simulink model "TST_ECBtn_VD"  (R2016b)
settings: Solver=FixedStepDiscrete  StartTime=0.0  StopTime=simTime  FixedStep=sampleTime  RelTol=1e-3
values from neighbouring files (symbols this model uses):
  testCase = 1    [initTST_ECBtn_VD_001.m]
libraries: simulink x4, UnitTest_Lib x2
settings Model: Creator=xinchangran  LastModifiedBy=xinchangran
settings DebuggingCC: SignalRangeChecking=error

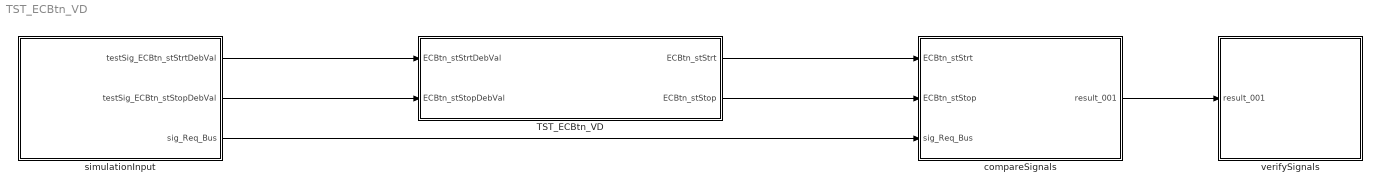
== system TST_ECBtn_VD ==
  TST_ECBtn_VD : Subsystem
  compareSignals : Subsystem
  simulationInput : Subsystem
  verifySignals : Subsystem
  wires:
  simulationInput/1(testSig_ECBtn_stStrtDebVal) -> TST_ECBtn_VD/1(ECBtn_stStrtDebVal)
  simulationInput/2(testSig_ECBtn_stStopDebVal) -> TST_ECBtn_VD/2(ECBtn_stStopDebVal)
  TST_ECBtn_VD/1(ECBtn_stStrt) -> compareSignals/1(ECBtn_stStrt)
  TST_ECBtn_VD/2(ECBtn_stStop) -> compareSignals/2(ECBtn_stStop)
  simulationInput/3(sig_Req_Bus) -> compareSignals/3(sig_Req_Bus)
  compareSignals/1(result_001) -> verifySignals/1(result_001)

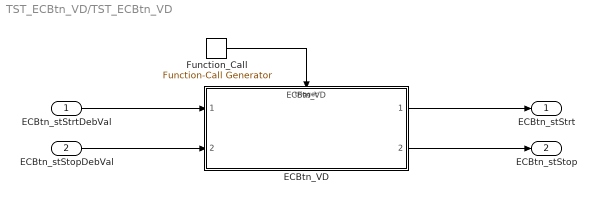
== system TST_ECBtn_VD/TST_ECBtn_VD ==
  ECBtn_stStrtDebVal : Inport
  ECBtn_stStopDebVal : Inport  Port=2
  ECBtn_VD : ModelReference  ModelNameDialog=ECBtn_VD  SimulationMode=Normal  ModelReferenceVersion=1.11  TriggerPortName=function  TriggerPortTriggerType=function-call  TriggerPortStatesWhenEnabling=held
  Function_Call : simulink/Ports & Subsystems/Function-Call Generator  sample_time=sampleTime  numberOfIterations=1
  ECBtn_stStrt : Outport
  ECBtn_stStop : Outport  Port=2
  wires:
  Function_Call/1 -> ECBtn_VD/Trigger
  ECBtn_stStrtDebVal/1 -> ECBtn_VD/1
  ECBtn_stStopDebVal/1 -> ECBtn_VD/2
  ECBtn_VD/1 -> ECBtn_stStrt/1
  ECBtn_VD/2 -> ECBtn_stStop/1

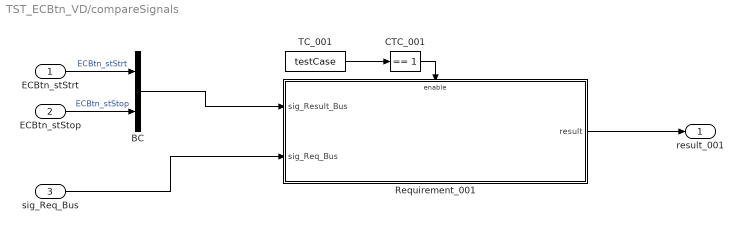
== system TST_ECBtn_VD/compareSignals ==
  ECBtn_stStrt : Inport
  ECBtn_stStop : Inport  Port=2
  sig_Req_Bus : Inport  Port=3
  BC : BusCreator  Inputs=2
  CTC_001 : simulink/Logic and Bit Operations/Compare To Constant  relop===  const=1  OutDataTypeStr=boolean
  Requirement_001 : Subsystem
  TC_001 : Constant  Value=testCase
  result_001 : Outport
  wires:
  ECBtn_stStrt/1 -> BC/1  "ECBtn_stStrt"
  ECBtn_stStop/1 -> BC/2  "ECBtn_stStop"
  TC_001/1 -> CTC_001/1
  CTC_001/1 -> Requirement_001/Enable
  sig_Req_Bus/1 -> Requirement_001/2(sig_Req_Bus)
  BC/1 -> Requirement_001/1(sig_Result_Bus)
  Requirement_001/1(result) -> result_001/1

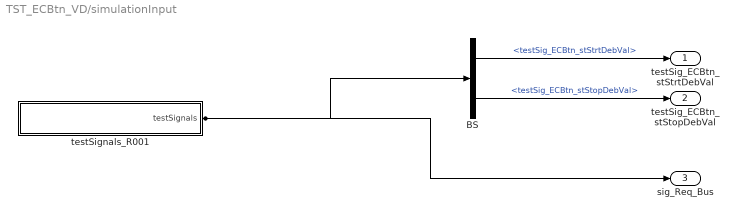
== system TST_ECBtn_VD/simulationInput ==
  BS : BusSelector  OutputSignals=testSig_ECBtn_stStrtDebVal,testSig_ECBtn_stStopDebVal
  testSignals_R001 : Subsystem
  testSig_ECBtn_stStrtDebVal : Outport
  testSig_ECBtn_stStopDebVal : Outport  Port=2
  sig_Req_Bus : Outport  Port=3
  wires:
  BS/1 -> testSig_ECBtn_stStrtDebVal/1  "<testSig_ECBtn_stStrtDebVal>"
  BS/2 -> testSig_ECBtn_stStopDebVal/1  "<testSig_ECBtn_stStopDebVal>"
  testSignals_R001/1(testSignals) -> BS/1, sig_Req_Bus/1

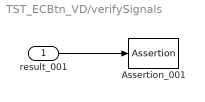
== system TST_ECBtn_VD/verifySignals ==
  result_001 : Inport
  Assertion_001 : Assertion  Enabled=off
  wires:
  result_001/1 -> Assertion_001/1

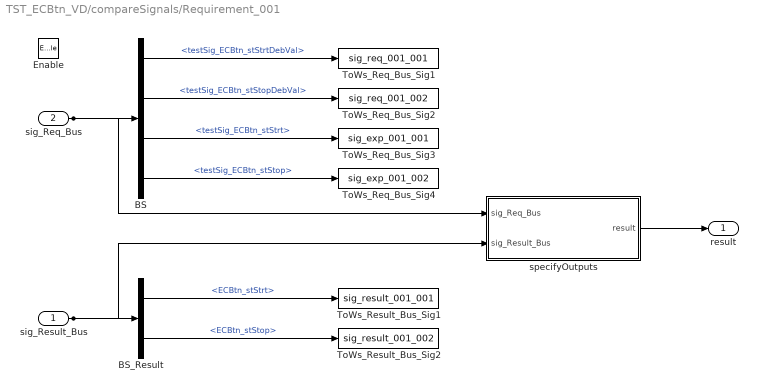
== system TST_ECBtn_VD/compareSignals/Requirement_001 ==
  sig_Result_Bus : Inport
  sig_Req_Bus : Inport  Port=2
  Enable : EnablePort
  BS : BusSelector  OutputSignals=testSig_ECBtn_stStrtDebVal,testSig_ECBtn_stStopDebVal,testSig_ECBtn_stStrt,testSig_ECBtn_stStop
  BS_Result : BusSelector  OutputSignals=ECBtn_stStrt,ECBtn_stStop
  ToWs_Req_Bus_Sig1 : ToWorkspace  VariableName=sig_req_001_001  SaveFormat=Structure With Time
  ToWs_Req_Bus_Sig2 : ToWorkspace  VariableName=sig_req_001_002  SaveFormat=Structure With Time
  ToWs_Req_Bus_Sig3 : ToWorkspace  VariableName=sig_exp_001_001  SaveFormat=Structure With Time
  ToWs_Req_Bus_Sig4 : ToWorkspace  VariableName=sig_exp_001_002  SaveFormat=Structure With Time
  ToWs_Result_Bus_Sig1 : ToWorkspace  VariableName=sig_result_001_001  SaveFormat=Structure With Time
  ToWs_Result_Bus_Sig2 : ToWorkspace  VariableName=sig_result_001_002  SaveFormat=Structure With Time
  specifyOutputs : Subsystem
  result : Outport
  wires:
  sig_Req_Bus/1 -> BS/1, specifyOutputs/1(sig_Req_Bus)
  BS/1 -> ToWs_Req_Bus_Sig1/1  "<testSig_ECBtn_stStrtDebVal>"
  BS/2 -> ToWs_Req_Bus_Sig2/1  "<testSig_ECBtn_stStopDebVal>"
  BS/3 -> ToWs_Req_Bus_Sig3/1  "<testSig_ECBtn_stStrt>"
  BS/4 -> ToWs_Req_Bus_Sig4/1  "<testSig_ECBtn_stStop>"
  sig_Result_Bus/1 -> BS_Result/1, specifyOutputs/2(sig_Result_Bus)
  BS_Result/1 -> ToWs_Result_Bus_Sig1/1  "<ECBtn_stStrt>"
  BS_Result/2 -> ToWs_Result_Bus_Sig2/1  "<ECBtn_stStop>"
  specifyOutputs/1(result) -> result/1

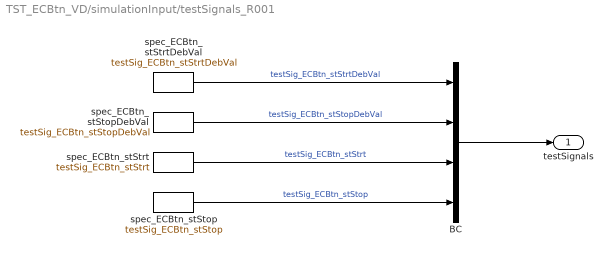
== system TST_ECBtn_VD/simulationInput/testSignals_R001 ==
  BC : BusCreator  Inputs=4
  spec_ECBtn_stStop : FromWorkspace  VariableName=testSig_ECBtn_stStop  Interpolate=off  OutputAfterFinalValue=Holding final value
  spec_ECBtn_stStopDebVal : FromWorkspace  VariableName=testSig_ECBtn_stStopDebVal  Interpolate=off  OutputAfterFinalValue=Holding final value
  spec_ECBtn_stStrt : FromWorkspace  VariableName=testSig_ECBtn_stStrt  Interpolate=off  OutputAfterFinalValue=Holding final value
  spec_ECBtn_stStrtDebVal : FromWorkspace  VariableName=testSig_ECBtn_stStrtDebVal  Interpolate=off  OutputAfterFinalValue=Holding final value
  testSignals : Outport
  wires:
  BC/1 -> testSignals/1
  spec_ECBtn_stStrtDebVal/1 -> BC/1  "testSig_ECBtn_stStrtDebVal"
  spec_ECBtn_stStopDebVal/1 -> BC/2  "testSig_ECBtn_stStopDebVal"
  spec_ECBtn_stStrt/1 -> BC/3  "testSig_ECBtn_stStrt"
  spec_ECBtn_stStop/1 -> BC/4  "testSig_ECBtn_stStop"

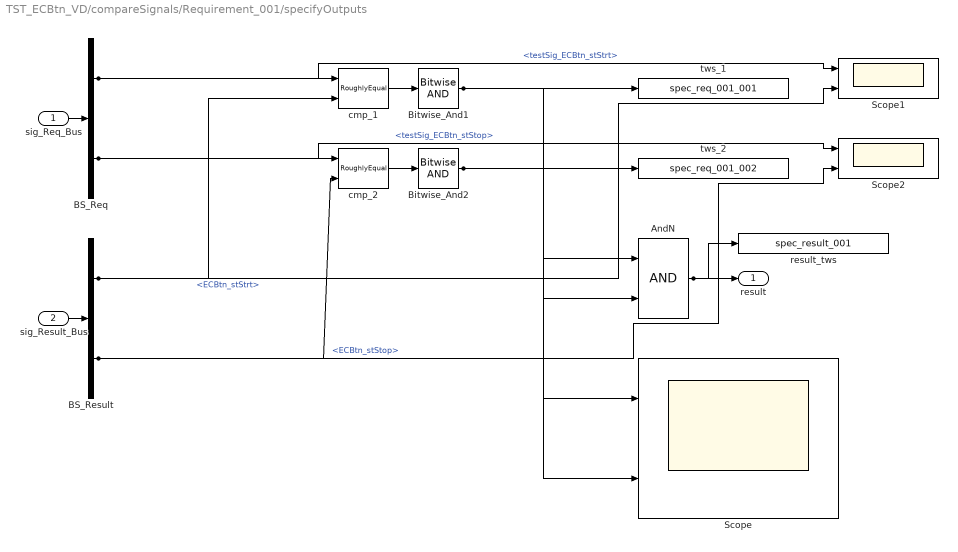
== system TST_ECBtn_VD/compareSignals/Requirement_001/specifyOutputs ==
  sig_Req_Bus : Inport
  sig_Result_Bus : Inport  Port=2
  AndN : Logic
  BS_Req : BusSelector  OutputSignals=testSig_ECBtn_stStrt,testSig_ECBtn_stStop
  BS_Result : BusSelector  OutputSignals=ECBtn_stStrt,ECBtn_stStop
  Bitwise_And1 : simulink/Logic and Bit Operations/Bitwise Operator  logicop=AND  UseBitMask=off  BitMask=bin2dec('11011001')  BitMaskRealWorld=Stored Integer
  Bitwise_And2 : simulink/Logic and Bit Operations/Bitwise Operator  logicop=AND  UseBitMask=off  BitMask=bin2dec('11011001')  BitMaskRealWorld=Stored Integer
  Scope : Scope  NumInputPorts=2
  Scope1 : Scope  NumInputPorts=2
  Scope2 : Scope  NumInputPorts=2
  cmp_1 : UnitTest_Lib/RoughlyEqual  slope=0.1
  cmp_2 : UnitTest_Lib/RoughlyEqual  slope=0.1
  result_tws : ToWorkspace  VariableName=spec_result_001
  tws_1 : ToWorkspace  VariableName=spec_req_001_001
  tws_2 : ToWorkspace  VariableName=spec_req_001_002
  result : Outport
  wires:
  sig_Req_Bus/1 -> BS_Req/1
  sig_Result_Bus/1 -> BS_Result/1
  AndN/1 -> result/1, result_tws/1
  BS_Req/1 -> cmp_1/1, Scope1/1  "<testSig_ECBtn_stStrt>"
  BS_Result/1 -> cmp_1/2, Scope1/2  "<ECBtn_stStrt>"
  cmp_1/1 -> Bitwise_And1/1
  Bitwise_And1/1 -> tws_1/1, AndN/1, Scope/1
  BS_Req/2 -> cmp_2/1, Scope2/1  "<testSig_ECBtn_stStop>"
  BS_Result/2 -> cmp_2/2, Scope2/2  "<ECBtn_stStop>"
  cmp_2/1 -> Bitwise_And2/1
  Bitwise_And2/1 -> tws_2/1, AndN/2, Scope/2
